simulink model "task1"  (R2015a)
settings: Solver=ode45  StartTime=0.0  StopTime=10.0  RelTol=1e-3
settings Model: Creator=Dell  LastModifiedBy=Dell

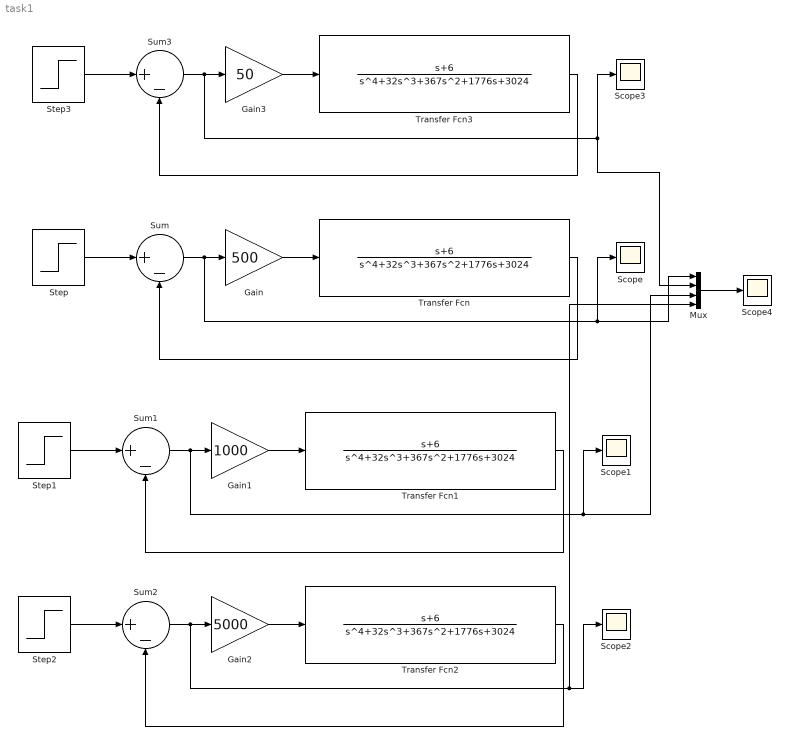
== system task1 ==
  Gain : Gain  Gain=500
  Gain1 : Gain  Gain=1000
  Gain2 : Gain  Gain=5000
  Gain3 : Gain  Gain=50
  Mux : Mux
  Scope{,1..4} (5 alike) : Scope
      Scope2 settings: SaveName=ScopeData2
      Scope3 settings: SaveName=ScopeData3
      Scope4 settings: SaveName=ScopeData4
  Step{,1..3} (4 alike) : Step  Time=5  SampleTime=0
  Sum{,1..3} (4 alike) : Sum  Inputs=|+-
  Transfer Fcn{,1..3} (4 alike) : TransferFcn  Numerator=[1, 6]  Denominator=|
      | [1, 32, 367, 1776, 3024
      | ]
  wires:
  Sum/1 -> Mux/1, Scope/1, Gain/1
  Step/1 -> Sum/1
  Gain/1 -> Transfer Fcn/1
  Transfer Fcn/1 -> Sum/2
  Sum1/1 -> Mux/3, Scope1/1, Gain1/1
  Step1/1 -> Sum1/1
  Gain1/1 -> Transfer Fcn1/1
  Transfer Fcn1/1 -> Sum1/2
  Sum2/1 -> Mux/4, Scope2/1, Gain2/1
  Step2/1 -> Sum2/1
  Gain2/1 -> Transfer Fcn2/1
  Transfer Fcn2/1 -> Sum2/2
  Sum3/1 -> Scope3/1, Mux/2, Gain3/1
  Step3/1 -> Sum3/1
  Gain3/1 -> Transfer Fcn3/1
  Transfer Fcn3/1 -> Sum3/2
  Mux/1 -> Scope4/1
